simulink model "ballOnWater"  (R2017b)
settings: Solver=FixedStepDiscrete  StartTime=0.0  StopTime=inf  FixedStep=1/50  RelTol=1e-3  EnableMultiTasking=on
PreLoadFcn:
  | BOW_startup
values from neighbouring files (symbols this model uses):
  K = Kext(1:6)    [BOW_startup.m]
  Rp = 4e-3    (= 0.004)    [BOW_startup.m]
undefined symbols (not defined in the file or in its folder): C, Dfilter, DiscIntNeverNeededParam, Discrete, F, G, Kd, Ki, KN, Kp, KR, P_const, P_offset, sat, Time
libraries: simulink x4, ctrlSharedLib x2, embdlinuxlib x1
settings Model: SimulationMode=external  Creator=Josef  LastModifiedBy=Josef
settings SolverCC: PositivePriorityOrder=on
settings OptimizationCC: PassReuseOutputArgsThreshold=0  MaxStackSize=64
settings DebuggingCC: ParameterTunabilityLossMsg=error
settings HardwareCC: ProdBitPerPointer=32  ProdBitPerSizeT=32  ProdBitPerPtrDiffT=32  ProdLargestAtomicInteger=Long  ProdLargestAtomicFloat=Double  ProdWordSize=32  ProdHWDeviceType=ARM Compatible->ARM Cortex  UseEmbeddedCoderFeatures=off
settings SFSimCC: MATLABDynamicMemAlloc=off
settings RTWCC: SystemTargetFile=ert.tlc  HardwareBoard=Raspberry Pi  TemplateMakefile=ert_default_tmf  GenerateReport=on  Toolchain=GNU GCC Raspberry Pi  TargetLang=C++
settings CodeAppCC: ForceParamTrailComments=on  OperatorAnnotations=on
settings ERTTargetCC: TargetLangStandard=C++03 (ISO)  ERTCustomFileBanners=off  SupportContinuousTime=on  SupportNonInlinedSFcns=on  RemoveResetFunc=off  SupportVariableSizeSignals=on  ModelStepFunctionPrototypeControlCompliant=off

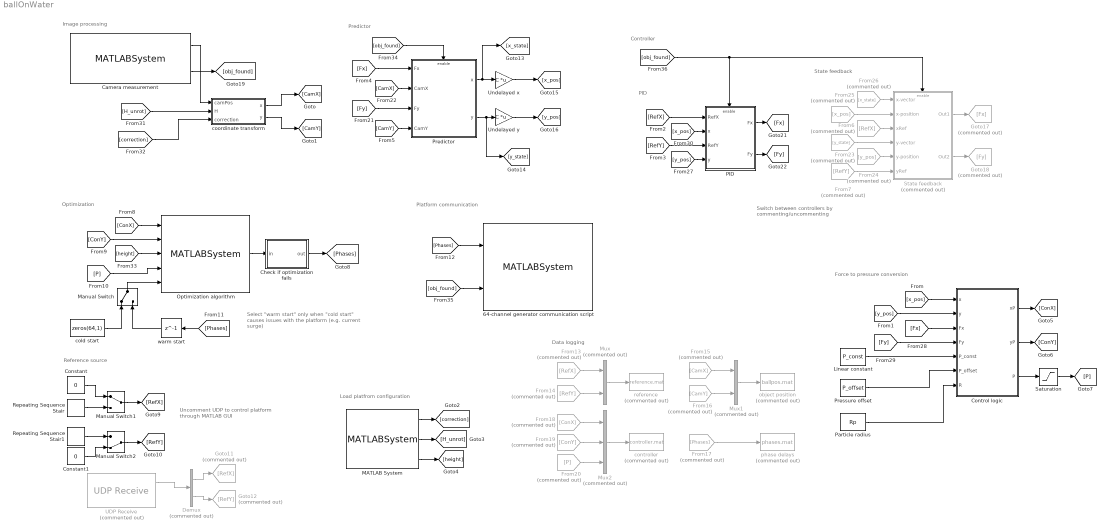
== system ballOnWater ==
  note: Load platfrom configuration
  note: Force to pressure conversion
  note: PID
  note: State feedback
  note: Uncomment UDP
      | to control platform
      | through MATLAB GUI
  note: Select "warm start" only when
      | "cold start" causes issues with
      | the platform (e.g. current surge)
  note: Switch between controllers by
      | commenting/uncommenting
  note: Data logging
  note: Reference source
  note: Platform communication
  note: Optimization
  note: Controller
  note: Image processing
  note: Predictor
  64-channel generator communication script : MATLABSystem  System=NewGenerator  Port=/dev/ttyUSB0  Baud=230400
      mask Type: NewGenerator
      mask Display:
      | disp(['64 phase generator' char(10) ' Port: /dev/ttyUSB0' char(10) ' Baudrate: 230400']);
      | port_label('input',1,'phases');
      | port_label('input',2,'On/Off');
  Camera measurement : MATLABSystem  System=RaspiBallPos  shm_key=3145914  framerate=50  N=1000  objects=1  km=eye( 3 )  notfound=0  execScript=off  concatenateOutputs=off  rotation=off  found_output=on
      mask Type: RaspiBallPos
      mask Display:
      | disp('RaspiBallPos');
      | port_label('output',1,'Position 1 [x;y]');
      | port_label('output',2,'Object found?');
  Check if optimization fails : MATLAB Function  TreatAsAtomicUnit=on
  Constant : Constant  Value=0
  Constant1 : Constant  Value=0
  Control logic : MATLAB Function  TreatAsAtomicUnit=on
  Demux : Demux  Commented=on  Outputs=2
  From13 : From  Commented=on  GotoTag=RefX
  From14 : From  Commented=on  GotoTag=RefY
  From15 : From  Commented=on  GotoTag=CamX
  From16 : From  Commented=on  GotoTag=CamY
  From17 : From  Commented=on  GotoTag=Phases
  From18 : From  Commented=on  GotoTag=ConX
  From19 : From  Commented=on  GotoTag=ConY
  From20 : From  Commented=on  GotoTag=P
  From23 : From  Commented=on  GotoTag=y_state
  From24 : From  Commented=on  GotoTag=y_pos
  From25 : From  Commented=on  GotoTag=x_pos
  From26 : From  Commented=on  GotoTag=x_state
  From6 : From  Commented=on  GotoTag=RefX
  From7 : From  Commented=on  GotoTag=RefY
  Goto11 : Goto  Commented=on  GotoTag=RefX
  Goto12 : Goto  Commented=on  GotoTag=RefY
  Goto17 : Goto  Commented=on  GotoTag=Fx
  Goto18 : Goto  Commented=on  GotoTag=Fy
  Linear constant : Constant  Value=P_const
  MATLAB System : MATLABSystem  System=Loader  corrFile=correction.bin  H_unFile=H_unrot.bin  heightFile=height.bin
      mask Type: Loader
      mask Display:
      | disp('Loader');
      | port_label('output',1,'correction');
      | port_label('output',2,'H_unrot');
      | port_label('output',3,'height');
  Manual Switch : ManualSwitch
  Manual Switch1 : ManualSwitch
  Manual Switch2 : ManualSwitch  CurrentSetting=0
  Mux : Mux  Commented=on  Inputs=2
  Mux1 : Mux  Commented=on  Inputs=2
  Mux2 : Mux  Commented=on  Inputs=3
  Optimization algorithm : MATLABSystem  System=PressurePoints
      mask Type: PressurePoints
      mask Display:
      | disp(['Pressure points' char(10) 'optimization']);
      | port_label('input',1,'x');
      | port_label('input',2,'y');
      | port_label('input',3,'z');
      | port_label('input',4,'Required pressure');
      | port_label('input',5,'Initial condition');
      | port_label('output',1,'Phases');
  PID : Subsystem
  Particle radius : Constant  Value=Rp
  Predictor : Subsystem
  Pressure offset : Constant  Value=P_offset
  Repeating Sequence Stair : simulink/Sources/Repeating Sequence Stair  OutValues=tx  tsamp=-1  OutMin=[]  OutMax=[]  OutDataTypeStr=double  OutputDataTypeScalingMode=double  OutDataType=fixdt(0,8)  ConRadixGroup=Best Precision: Vector-wise  OutScaling=2^-12
  Repeating Sequence Stair1 : simulink/Sources/Repeating Sequence Stair  OutValues=ty  tsamp=-1  OutMin=[]  OutMax=[]  OutDataTypeStr=double  OutputDataTypeScalingMode=double  OutDataType=fixdt(0,8)  ConRadixGroup=Best Precision: Vector-wise  OutScaling=2^-12
  Saturation : Saturate  UpperLimit=2500  LowerLimit=0
  State feedback : Subsystem  Commented=on
  UDP Receive : embdlinuxlib/UDP Receive  Commented=on  localURL='0.0.0.0'  localPort=25000  remoteURL='0.0.0.0'  remotePort=-1  recvBufferSize=8192  signalDatatype=double  dims=2  isVarSize=off  showBlockingTime=off  blockingTime=0  sampletime=1/50  blockPlatform=Raspberry Pi
      settings: SourceProductName=Simulink Support Package for Raspberry Pi Hardware  SourceProductBaseCode=RASPPI
  Undelayed x : Gain  Gain=C  Multiplication=Matrix(K*u)
  Undelayed y : Gain  Gain=C  Multiplication=Matrix(K*u)
  cold start : Constant  Value=zeros(64,1)
  controller : ToFile  Commented=on  Filename=controller.mat  MatrixName=controller
  coordinate transform : MATLAB Function  TreatAsAtomicUnit=on
  object position : ToFile  Commented=on  Filename=ballpos.mat  MatrixName=ballpos
  phase delays : ToFile  Commented=on  Filename=phases.mat  MatrixName=phases
  reference : ToFile  Commented=on  Filename=reference.mat  MatrixName=ref
  warm start : Delay  DelayLength=1  InitialCondition=zeros(64,1)
  wires:
  coordinate transform/1(x) -> [CamX]
  [H_unrot] -> coordinate transform/2(H)
  coordinate transform/2(y) -> [CamY]
  Camera measurement/1 -> coordinate transform/1(camPos)
  [correction] -> coordinate transform/3(correction)
  Check if optimization fails/1(out) -> [Phases]
  [ConX] -> Optimization algorithm/1
  [ConY] -> Optimization algorithm/2
  [Phases] -> warm start/1
  [P] -> Optimization algorithm/4
  Optimization algorithm/1 -> Check if optimization fails/1(in)
  cold start/1 -> Manual Switch/1
  warm start/1 -> Manual Switch/2
  Manual Switch/1 -> Optimization algorithm/5
  [height] -> Optimization algorithm/3
  [Phases] -> 64-channel generator communication script/1
  [obj_found] -> 64-channel generator communication script/2
  UDP Receive/1 -> Demux/1
  Demux/1 -> Goto11/1
  Demux/2 -> Goto12/1
  Manual Switch2/1 -> [RefY]
  Manual Switch1/1 -> [RefX]
  From13/1 -> Mux/1
  From15/1 -> Mux1/1
  Mux1/1 -> object position/1
  From16/1 -> Mux1/2
  From18/1 -> Mux2/1
  From20/1 -> Mux2/3
  From19/1 -> Mux2/2
  Mux/1 -> reference/1
  From14/1 -> Mux/2
  From17/1 -> phase delays/1
  Mux2/1 -> controller/1
  Constant/1 -> Manual Switch1/1
  Constant1/1 -> Manual Switch2/2
  Repeating Sequence Stair/1 -> Manual Switch1/2
  Repeating Sequence Stair1/1 -> Manual Switch2/1
  Undelayed x/1 -> [x_pos]
  Undelayed y/1 -> [y_pos]
  [Fy] -> Control logic/4(Fy)
  [x_pos] -> Control logic/1(x)
  [Fx] -> Control logic/3(Fx)
  [y_pos] -> Control logic/2(y)
  Control logic/3(P) -> Saturation/1
  Pressure offset/1 -> Control logic/6(P_offset)
  Particle radius/1 -> Control logic/7(R)
  Linear constant/1 -> Control logic/5(P_const)
  Control logic/1(xP) -> [ConX]
  Control logic/2(yP) -> [ConY]
  Saturation/1 -> [P]
  MATLAB System/3 -> [height]
  MATLAB System/2 -> [H_unrot]
  MATLAB System/1 -> [correction]
  Predictor/1(x) -> [x_state], Undelayed x/1
  Predictor/2(y) -> [y_state], Undelayed y/1
  [Fx] -> Predictor/1(Fx)
  [CamX] -> Predictor/2(CamX)
  [Fy] -> Predictor/3(Fy)
  [CamY] -> Predictor/4(CamY)
  Camera measurement/2 -> [obj_found]
  [obj_found] -> Predictor/Enable
  [RefX] -> PID/1(RefX)
  [x_pos] -> PID/2(x)
  [RefY] -> PID/3(RefY)
  [y_pos] -> PID/4(y)
  PID/1(Fx) -> [Fx]
  PID/2(Fy) -> [Fy]
  From26/1 -> State feedback/1(x-vector)
  From25/1 -> State feedback/2(x-position)
  From6/1 -> State feedback/3(xRef)
  From7/1 -> State feedback/6(yRef)
  From24/1 -> State feedback/5(y-position)
  From23/1 -> State feedback/4(y-vector)
  State feedback/1(Out1) -> Goto17/1
  State feedback/2(Out2) -> Goto18/1
  [obj_found] -> State feedback/Enable, PID/Enable

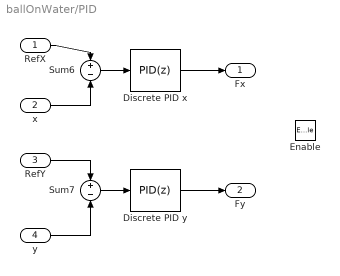
== system ballOnWater/PID ==
  RefX : Inport
  x : Inport  Port=2
  RefY : Inport  Port=3
  y : Inport  Port=4
  Enable : EnablePort  StatesWhenEnabling=reset
  Discrete PID x : simulink/Continuous/PID Controller  Controller=PID  TimeDomain=Discrete-time  SampleTime=-1  IntegratorMethod=Forward Euler  FilterMethod=Forward Euler  Form=Parallel  UseFilter=on  ControllerParametersSource=internal  P=Kp  I=Ki  D=Kd  N=Dfilter  InitialConditionSource=internal  InitialConditionForIntegrator=0  InitialConditionForFilter=0  ExternalReset=none  LimitOutput=on  UpperSaturationLimit=sat  LowerSaturationLimit=-sat  LinearizeAsGain=off  AntiWindupMode=clamping  Kb=1  TrackingMode=off  Kt=1  PParamMin=[]  PParamMax=[]  IParamMin=[]  IParamMax=[]  DParamMin=[]  DParamMax=[]  NParamMin=[]  NParamMax=[]  KbParamMin=[]  KbParamMax=[]  KtParamMin=[]  KtParamMax=[]  POutMin=[]  POutMax=[]  IOutMin=[]  IOutMax=[]  DOutMin=[]  DOutMax=[]  NOutMin=[]  NOutMax=[]  KbOutMin=[]  KbOutMax=[]  KtOutMin=[]  KtOutMax=[]  IntegratorOutMin=[]  IntegratorOutMax=[]  FilterOutMin=[]  FilterOutMax=[]  SumOutMin=[]  SumOutMax=[]  SumI1OutMin=[]  SumI1OutMax=[]  SumI2OutMin=[]  SumI2OutMax=[]  SumI3OutMin=[]  SumI3OutMax=[]  SumDOutMin=[]  SumDOutMax=[]  SaturationOutMin=[]  SaturationOutMax=[]  IntegratorContinuousStateAttributes=''  IntegratorStateMustResolveToSignalObject=off  IntegratorRTWStateStorageClass=Auto  FilterContinuousStateAttributes=''  FilterStateMustResolveToSignalObject=off  FilterRTWStateStorageClass=Auto  DifferentiatorICPrevScaledInput=0  DifferentiatorOutMin=[]  DifferentiatorOutMax=[]  InitialConditionSetting=State (most efficient)  FilterDiffOutCoefMin=[]  FilterDiffOutCoefMax=[]  SumDenOutMin=[]  SumDenOutMax=[]  SumNumOutMin=[]  SumNumOutMax=[]  ReciprocalOutMin=[]  ReciprocalOutMax=[]  DivideOutMin=[]  DivideOutMax=[]  TunerSelectOption=Transfer Function Based (PID Tuner App)
  Discrete PID y : simulink/Continuous/PID Controller  Controller=PID  TimeDomain=Discrete-time  SampleTime=-1  IntegratorMethod=Forward Euler  FilterMethod=Forward Euler  Form=Parallel  UseFilter=on  ControllerParametersSource=internal  P=Kp  I=Ki  D=Kd  N=Dfilter  InitialConditionSource=internal  InitialConditionForIntegrator=0  InitialConditionForFilter=0  ExternalReset=none  LimitOutput=on  UpperSaturationLimit=sat  LowerSaturationLimit=-sat  LinearizeAsGain=off  AntiWindupMode=clamping  Kb=1  TrackingMode=off  Kt=1  PParamMin=[]  PParamMax=[]  IParamMin=[]  IParamMax=[]  DParamMin=[]  DParamMax=[]  NParamMin=[]  NParamMax=[]  KbParamMin=[]  KbParamMax=[]  KtParamMin=[]  KtParamMax=[]  POutMin=[]  POutMax=[]  IOutMin=[]  IOutMax=[]  DOutMin=[]  DOutMax=[]  NOutMin=[]  NOutMax=[]  KbOutMin=[]  KbOutMax=[]  KtOutMin=[]  KtOutMax=[]  IntegratorOutMin=[]  IntegratorOutMax=[]  FilterOutMin=[]  FilterOutMax=[]  SumOutMin=[]  SumOutMax=[]  SumI1OutMin=[]  SumI1OutMax=[]  SumI2OutMin=[]  SumI2OutMax=[]  SumI3OutMin=[]  SumI3OutMax=[]  SumDOutMin=[]  SumDOutMax=[]  SaturationOutMin=[]  SaturationOutMax=[]  IntegratorContinuousStateAttributes=''  IntegratorStateMustResolveToSignalObject=off  IntegratorRTWStateStorageClass=Auto  FilterContinuousStateAttributes=''  FilterStateMustResolveToSignalObject=off  FilterRTWStateStorageClass=Auto  DifferentiatorICPrevScaledInput=0  DifferentiatorOutMin=[]  DifferentiatorOutMax=[]  InitialConditionSetting=State (most efficient)  FilterDiffOutCoefMin=[]  FilterDiffOutCoefMax=[]  SumDenOutMin=[]  SumDenOutMax=[]  SumNumOutMin=[]  SumNumOutMax=[]  ReciprocalOutMin=[]  ReciprocalOutMax=[]  DivideOutMin=[]  DivideOutMax=[]  TunerSelectOption=Frequency Response Based
  Sum6 : Sum  Inputs=+-
  Sum7 : Sum  Inputs=+-
  Fx : Outport
  Fy : Outport  Port=2
  wires:
  RefX/1 -> Sum6/1
  Sum6/1 -> Discrete PID x/1
  x/1 -> Sum6/2
  y/1 -> Sum7/2
  Discrete PID x/1 -> Fx/1
  RefY/1 -> Sum7/1
  Discrete PID y/1 -> Fy/1
  Sum7/1 -> Discrete PID y/1

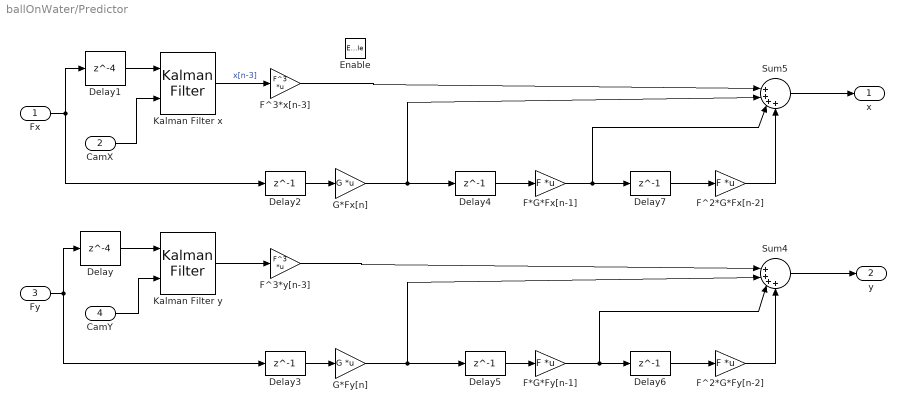
== system ballOnWater/Predictor ==
  Fx : Inport
  CamX : Inport  Port=2
  Fy : Inport  Port=3
  CamY : Inport  Port=4
  Enable : EnablePort  StatesWhenEnabling=reset
  Delay : Delay  DelayLength=4
  Delay1 : Delay  DelayLength=4
  Delay{2..7} (6 alike) : Delay  DelayLength=1
  F*G*Fx[n-1] : Gain  Gain=F  Multiplication=Matrix(K*u)
  F*G*Fy[n-1] : Gain  Gain=F  Multiplication=Matrix(K*u)
  F^2*G*Fx[n-2] : Gain  Gain=F  Multiplication=Matrix(K*u)
  F^2*G*Fy[n-2] : Gain  Gain=F  Multiplication=Matrix(K*u)
  F^3*x[n-3] : Gain  Gain=F^3  Multiplication=Matrix(K*u)
  F^3*y[n-3] : Gain  Gain=F^3  Multiplication=Matrix(K*u)
  G*Fx[n] : Gain  Gain=G  Multiplication=Matrix(K*u)
  G*Fy[n] : Gain  Gain=G  Multiplication=Matrix(K*u)
  Kalman Filter x : ctrlSharedLib/Kalman Filter  TimeDomain=Discrete-Time  UseCurrentEstimator=on  ModelSource=Individual A, B, C, D matrices  ModelSourceVariable=ss(0.95,1,1,0,1)  A=F  B=G  C=C  D=0  NumberOfStates=1  NumberOfInputs=1  NumberOfOutputs=1  InitialEstimateSource=Dialog  X0=0  P0=10  UseK=off  UseGH=off  NumberOfProcessNoiseInputs=1  G=1  TimeInvariantG=on  H=0  TimeInvariantH=on  Q=KQ  TimeInvariantQ=on  R=KR  TimeInvariantR=on  N=KN  TimeInvariantN=on  AddInputPort=on  AddEnablePort=off  OutputEstimatedY=off  OutputP=off  Ts=1/50
      settings: SourceProductBaseCode=CT
  Kalman Filter y : ctrlSharedLib/Kalman Filter  TimeDomain=Discrete-Time  UseCurrentEstimator=on  ModelSource=Individual A, B, C, D matrices  ModelSourceVariable=ss(0.95,1,1,0,1)  A=F  B=G  C=C  D=0  NumberOfStates=1  NumberOfInputs=1  NumberOfOutputs=1  InitialEstimateSource=Dialog  X0=0  P0=10  UseK=off  UseGH=off  NumberOfProcessNoiseInputs=1  G=1  TimeInvariantG=on  H=0  TimeInvariantH=on  Q=KQ  TimeInvariantQ=on  R=KR  TimeInvariantR=on  N=KN  TimeInvariantN=on  AddInputPort=on  AddEnablePort=off  OutputEstimatedY=off  OutputP=off  Ts=1/50
      settings: SourceProductBaseCode=CT
  Sum4 : Sum  Inputs=||++++
  Sum5 : Sum  Inputs=||++++
  x : Outport
  y : Outport  Port=2
  wires:
  Fx/1 -> Delay1/1, Delay2/1
  G*Fy[n]/1 -> Sum4/2, Delay5/1
  Delay1/1 -> Kalman Filter x/1
  Delay/1 -> Kalman Filter y/1
  CamX/1 -> Kalman Filter x/2
  Kalman Filter x/1 -> F^3*x[n-3]/1  "x[n-3]"
  Kalman Filter y/1 -> F^3*y[n-3]/1
  Delay3/1 -> G*Fy[n]/1
  CamY/1 -> Kalman Filter y/2
  Fy/1 -> Delay/1, Delay3/1
  F^3*x[n-3]/1 -> Sum5/1
  Sum4/1 -> y/1
  F*G*Fy[n-1]/1 -> Sum4/3, Delay6/1
  Delay6/1 -> F^2*G*Fy[n-2]/1
  G*Fx[n]/1 -> Sum5/2, Delay4/1
  F^3*y[n-3]/1 -> Sum4/1
  Delay5/1 -> F*G*Fy[n-1]/1
  Delay7/1 -> F^2*G*Fx[n-2]/1
  F^2*G*Fx[n-2]/1 -> Sum5/4
  F^2*G*Fy[n-2]/1 -> Sum4/4
  F*G*Fx[n-1]/1 -> Delay7/1, Sum5/3
  Delay2/1 -> G*Fx[n]/1
  Delay4/1 -> F*G*Fx[n-1]/1
  Sum5/1 -> x/1

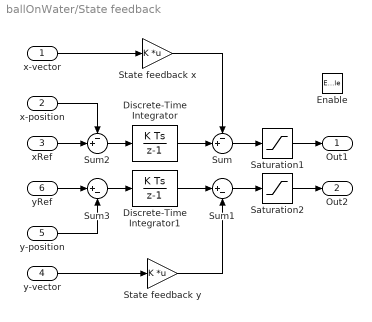
== system ballOnWater/State feedback ==
  x-vector : Inport
  x-position : Inport  Port=2
  xRef : Inport  Port=3
  y-vector : Inport  Port=4
  y-position : Inport  Port=5
  yRef : Inport  Port=6
  Enable : EnablePort
  Discrete-Time Integrator : DiscreteIntegrator  gainval=K_i  InitialConditionSetting=State (most efficient)  SampleTime=1/50  UpperSaturationLimit=sat  LowerSaturationLimit=-sat  ICPrevOutput=DiscIntNeverNeededParam  ICPrevScaledInput=DiscIntNeverNeededParam
  Discrete-Time Integrator1 : DiscreteIntegrator  gainval=K_i  InitialConditionSetting=State (most efficient)  SampleTime=1/50  UpperSaturationLimit=sat  LowerSaturationLimit=-sat  ICPrevOutput=DiscIntNeverNeededParam  ICPrevScaledInput=DiscIntNeverNeededParam
  Saturation1 : Saturate  UpperLimit=sat  LowerLimit=-sat
  Saturation2 : Saturate  UpperLimit=sat  LowerLimit=-sat
  State feedback x : Gain  Gain=K  Multiplication=Matrix(K*u)
  State feedback y : Gain  Gain=K  Multiplication=Matrix(K*u)
  Sum : Sum  Inputs=-+|
  Sum1 : Sum  Inputs=|+-
  Sum2 : Sum  Inputs=-+|
  Sum3 : Sum  Inputs=|+-
  Out1 : Outport
  Out2 : Outport  Port=2
  wires:
  State feedback y/1 -> Sum1/2
  Discrete-Time Integrator1/1 -> Sum1/1
  Discrete-Time Integrator/1 -> Sum/2
  Sum2/1 -> Discrete-Time Integrator/1
  State feedback x/1 -> Sum/1
  Sum3/1 -> Discrete-Time Integrator1/1
  xRef/1 -> Sum2/2
  y-position/1 -> Sum3/2
  Sum1/1 -> Saturation2/1
  x-position/1 -> Sum2/1
  y-vector/1 -> State feedback y/1
  yRef/1 -> Sum3/1
  x-vector/1 -> State feedback x/1
  Sum/1 -> Saturation1/1
  Saturation1/1 -> Out1/1
  Saturation2/1 -> Out2/1

== matlab function ballOnWater/coordinate transform ==
  data: x output; camPos input; y output; H input; correction input
function [x,y] = trans(camPos, H, correction)
    [x,y] = coordTransform(H, camPos, correction);
end

== matlab function ballOnWater/Check if optimization fails ==
  data: in input; out output
function out = NaNcontrol(in)
    if isnan(in)
        out = zeros(64,1);
    else
        out = in;
    end
% % end

== matlab function ballOnWater/Control logic ==
  data: x input; xP output; y input; Fx input; Fy input; P_const input; P_offset input; R input; yP output; P output
function [xP,yP,P] = forceToPressure(x,y,Fx,Fy,P_const,P_offset,R)    
    F = sqrt(Fx^2 + Fy^2);
    P = P_const*F + P_offset;
    cosA = Fx/F;
    sinA = Fy/F;
    xP = x - (R+0.0015)*cosA;
    yP = y - (R+0.0015)*sinA;
end
